simulink model "ThreePhaseFullyControlledDCMachine"  (R2024b)
settings: Solver=VariableStepAuto  StartTime=0.0  StopTime=0.1  RelTol=1e-3
libraries: spsThyristorLib x6, spsVoltageMeasurementLib x4, spsDCMachineLib x1, spsDCVoltageSourceLib x1, spsGroundLib x1, spsThreePhaseProgrammableVoltageSourceLib x1, sps_lib x1
settings Model: Creator=harsh  LastModifiedBy=hp

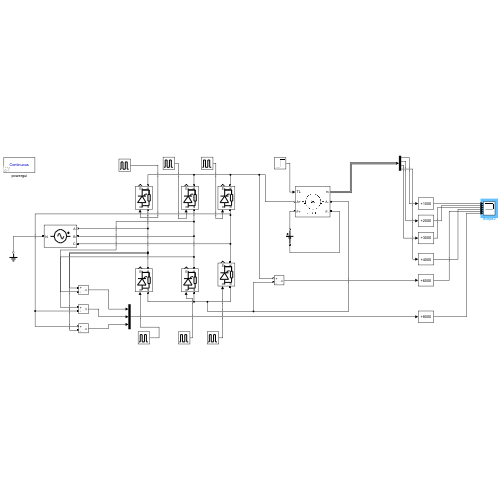
[thumbnail: Simulink's stored preview of the top-level diagram]
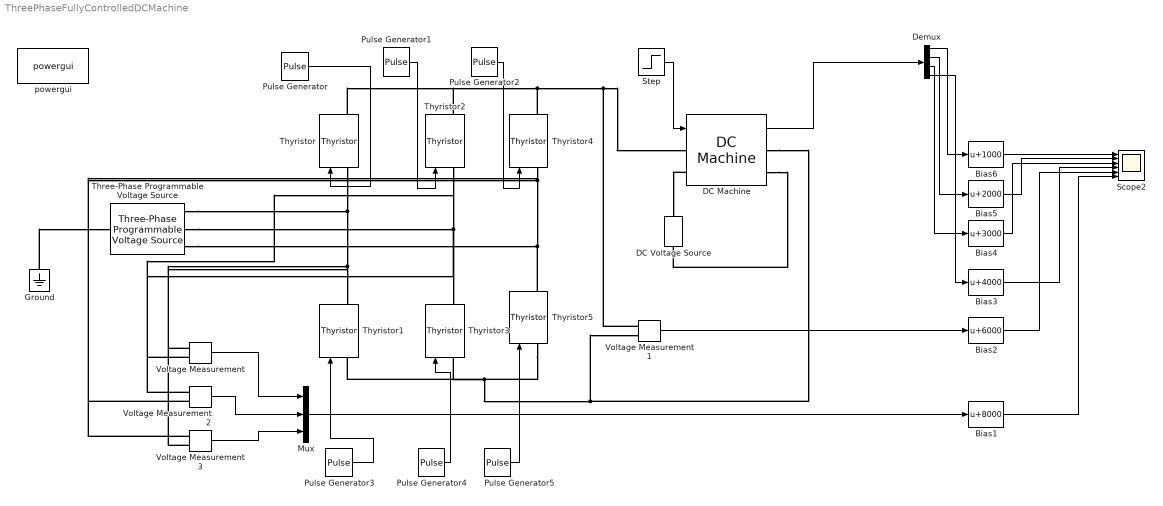
== system ThreePhaseFullyControlledDCMachine ==
  Bias1 : Bias  Bias=8000  SaturateOnIntegerOverflow=off
  Bias2 : Bias  Bias=6000  SaturateOnIntegerOverflow=off
  Bias3 : Bias  Bias=4000  SaturateOnIntegerOverflow=off
  Bias4 : Bias  Bias=3000  SaturateOnIntegerOverflow=off
  Bias5 : Bias  Bias=2000  SaturateOnIntegerOverflow=off
  Bias6 : Bias  Bias=1000  SaturateOnIntegerOverflow=off
  DC Machine : spsDCMachineLib/DC Machine  PresetModel=No  MechanicalLoad=Torque TL  FieldType=Wound  ShowDetailedParameters=on  MeasurementBus=off  RLa="[ 0.6  0.012]"  RLf="[ 240  120]"  Laf=1.8  MachineConstant=Torque constant (N.m/A)  Ke=1.8  Kt=1.8  J=1  Bm=0  Tf=0  w0=1  Ifinit=0.416666666255433  TsPowergui=0  TsBlock=-1
  DC Voltage Source : spsDCVoltageSourceLib/DC Voltage Source  Amplitude=100  Measurements=None
  Demux : Demux
  Ground : spsGroundLib/Ground  LConnTagsString=a
  Mux : Mux  Inputs=3
  Pulse Generator : DiscretePulseGenerator  PulseType=Time based  Period=0.02  PulseWidth=5  PhaseDelay=0*0.02/360
  Pulse Generator1 : DiscretePulseGenerator  PulseType=Time based  Period=0.02  PulseWidth=5  PhaseDelay=(0+120)*0.02/360
  Pulse Generator2 : DiscretePulseGenerator  PulseType=Time based  Period=0.02  PulseWidth=5  PhaseDelay=(0+240)*0.02/360
  Pulse Generator3 : DiscretePulseGenerator  PulseType=Time based  Period=0.02  PulseWidth=5  PhaseDelay=(0+180)*0.02/360
  Pulse Generator4 : DiscretePulseGenerator  PulseType=Time based  Period=0.02  PulseWidth=5  PhaseDelay=(0+300)*0.02/360
  Pulse Generator5 : DiscretePulseGenerator  PulseType=Time based  Period=0.02  PulseWidth=5  PhaseDelay=(0+60)*0.02/360
  Scope2 : Scope  NumInputPorts=6
  Step : Step  SampleTime=0
  Three-Phase Programmable Voltage Source : spsThreePhaseProgrammableVoltageSourceLib/Three-Phase Programmable Voltage Source  PositiveSequence="[415  0 50]"  VariationEntity=None  VariationType=Table of time-amplitude pairs  VariationTypeAlt=Step  VariationStep=0.5  VariationRate=10  VariationMagnitude=0.3  VariationFrequency=2  VariationTiming=[1 2]  VariationPhaseA=off  Amplitudes=[1 0.8 1.2 1.0]  TimeValues=[0 0.1 0.15 0.2]  HarmonicGeneration=off  HarmonicA=[3 0.2 -25 0]  HarmonicB=[2 0.15 35 2]  Timing="[0.05  3]"  BusType=swing  Pref=0  Qref=0  Qmin=-inf  Qmax=inf
  Thyristor{,1..5} (6 alike) : spsThyristorLib/Thyristor  Ron=0.001  Lon=0  Vf=0.8  IC=0  Rs=500  Cs=250e-9  Measurements=on
  Voltage Measurement{,1..3} (4 alike) : spsVoltageMeasurementLib/Voltage Measurement  PhasorSimulation=off  OutputType=Complex  PSBequivalent=0
  powergui : sps_lib/powergui  Priority=1  SimulationMode=Continuous  SampleTime=50e-6  frequency=60  Iterations=50  frequencyindice=50  Pbase=100e6  ErrMax=1e-4  UnitsV=kV  UnitsW=MW  buscounter=0  FunctionMessages=off  echomessages=off  EnableUseOfTLC=off  CurrentSourceSwitches=off  DisableSnubberDevices=off  DisableRonSwitches=off  DisableVfSwitches=off  DisplayEquations=off  AutomaticDiscreteSolvers=off  SolverType=Tustin/Backward Euler (TBE)  Interpol=off  ExternalGateDelay=off  methode=off  Ts=100  x0status=blocks  SPID=on  SwTol=0  HookPort=off  NonlinearTolerance=1e-4  nMaxIteration=100  ContinueOnMaxIteration=off  RestoreLinks=warning  ResistiveCurrentMeasurement=off  Frange=[0:2:500]  Ylog=off  Xlog=on  ShowGrid=off  save=off  variable=ZData  structure=0  ZoomFFT=off  StartTime=0.0  cycles=1  DisplayStyle=1  fundamental=60  FreqAxis=off  MaxFrequency=1000  frequencyindicesteady=1  RmsSteady=1  display=off
  wires:
  Pulse Generator1/1 -> Thyristor2/1
  Pulse Generator2/1 -> Thyristor4/1
  Pulse Generator/1 -> Thyristor/1
  Step/1 -> DC Machine/1
  Voltage Measurement/1 -> Mux/1
  Voltage Measurement2/1 -> Mux/2
  Voltage Measurement3/1 -> Mux/3
  Mux/1 -> Bias1/1
  Voltage Measurement1/1 -> Bias2/1
  DC Machine/1 -> Demux/1
  Bias1/1 -> Scope2/6
  Bias2/1 -> Scope2/5
  Demux/1 -> Bias6/1
  Demux/2 -> Bias5/1
  Demux/3 -> Bias4/1
  Demux/4 -> Bias3/1
  Bias6/1 -> Scope2/1
  Bias5/1 -> Scope2/2
  Bias4/1 -> Scope2/3
  Bias3/1 -> Scope2/4
  Pulse Generator3/1 -> Thyristor1/1
  Pulse Generator4/1 -> Thyristor3/1
  Pulse Generator5/1 -> Thyristor5/1
  connections:
  Thyristor1/LConn1 -- Thyristor3/LConn1 -- Thyristor5/LConn1 -- DC Machine/RConn1 -- Voltage Measurement1/LConn2
  Voltage Measurement1/LConn1 -- DC Machine/LConn1 -- Thyristor4/RConn1 -- Thyristor2/RConn1 -- Thyristor/RConn1
  Thyristor/LConn1 -- Three-Phase Programmable Voltage Source/RConn1 -- Thyristor1/RConn1 -- Voltage Measurement3/LConn2 -- Voltage Measurement/LConn1
  Three-Phase Programmable Voltage Source/RConn2 -- Voltage Measurement2/LConn1 -- Thyristor3/RConn1 -- Thyristor2/LConn1 -- Voltage Measurement/LConn2
  Thyristor4/LConn1 -- Voltage Measurement3/LConn1 -- Voltage Measurement2/LConn2 -- Thyristor5/RConn1 -- Three-Phase Programmable Voltage Source/RConn3
  Ground/LConn1 -- Three-Phase Programmable Voltage Source/LConn1
  DC Machine/LConn2 -- DC Voltage Source/RConn1
  DC Machine/RConn2 -- DC Voltage Source/LConn1
